simulink model "receiver_overall_v3"  (Simulink 7.5)
settings: Solver=FixedStepDiscrete  SolverMode=SingleTasking  StartTime=0.0  StopTime=(length(simin.signals.values)-1)/Fs  FixedStep=1  RelTol=1e-3
undefined symbols (not defined in the file): Fs
libraries: xbsIndex_r4 x939, symbols x8, dspsigops x2
(part 5 of 9)

== system receiver_overall_v3/Receiver/FM demod/AGC/CORDIC DIVIDER/Iterative Divider/CORDIC PE7 ==
  note: X = x - y if y < 0, otherwise
      |    = x + y
      | Y = y + x if y < 0, otherwise
      |    = y - x
      | Z = z - atan(1/2^i) if y < 0, otherwise
      |    = z + atan(1/2^i)
  x : Inport  OutDataType=sfix(16)  OutScaling=2^0
  y : Inport  Port=2  OutDataType=sfix(16)  OutScaling=2^0
  z : Inport  Port=3  OutDataType=sfix(16)  OutScaling=2^0
  AddSub1 : xbsIndex_r4/AddSub  mode=Addition or Subtraction  use_carryin=off  use_carryout=off  en=off  latency=pipeline  precision=User Defined  arith_type="Signed  (2's comp)"  n_bits=pe_nbits  bin_pt=pe_binpt  quantization=Truncate  overflow=Wrap  dbl_ovrd=off  use_behavioral_HDL=on  hw_selection=Fabric  pipelined=off  use_rpm=off  block_type=addsub
      settings: xl_area=[8 16 0 16 0 0 0]  block_version=VER_STRING_GOES_HERE
  AddSub2 : xbsIndex_r4/AddSub  mode=Addition or Subtraction  use_carryin=off  use_carryout=off  en=off  latency=pipeline  precision=User Defined  arith_type="Signed  (2's comp)"  n_bits=stages+2  bin_pt=stages  quantization=Truncate  overflow=Wrap  dbl_ovrd=off  use_behavioral_HDL=on  hw_selection=Fabric  pipelined=off  use_rpm=off  block_type=addsub
      settings: xl_area=[8 16 0 16 0 0 0]  block_version=VER_STRING_GOES_HERE
  Constant : xbsIndex_r4/Constant  arith_type=Signed (2's comp)  const=2^-ii  n_bits=stages+2  bin_pt=stages  explicit_period=off  period=1  equ=P=C  opselect=C  inp2=PCIN>>17  opr=+  inp1=P  carry=CIN  dbl_ovrd=off  block_type=constant
      settings: block_version=VER_STRING_GOES_HERE
  Inverter : xbsIndex_r4/Inverter  en=off  latency=0  dbl_ovrd=off  block_type=inv
      settings: xl_area=[1 0 0 1 0 0 0]  block_version=VER_STRING_GOES_HERE
  Register : xbsIndex_r4/Register  init=0  rst=off  en=off  dbl_ovrd=off  block_type=register
      settings: xl_area=[8 16 0 0 0 0 0]  block_version=VER_STRING_GOES_HERE
  Shift : xbsIndex_r4/Shift  shift_dir=Right  shift_bits=ii  en=off  latency=0  precision=User Defined  arith_type="Signed  (2's comp)"  n_bits=pe_nbits  bin_pt=pe_binpt  quantization=Truncate  overflow=Wrap  dbl_ovrd=off  block_type=shift
      settings: xl_area=[0 0 0 0 0 0 0]  block_version=VER_STRING_GOES_HERE
  Slice : xbsIndex_r4/Slice  nbits=1  boolean_output=on  mode=Upper Bit Location + Width  bit1=0  base1=MSB of Input  bit0=0  base0=LSB of Input  dbl_ovrd=off  block_type=slice
      settings: infoedit="Extracts a given range of bits from each input sample and presents it at the output.  The output type is ordinarily unsigned with binary point at zero, but can be Boolean when the slice is one bit wide.<P><P>Hardware notes: In hardware this block costs nothing."  block_version=VER_STRING_GOES_HERE
  X : Outport  OutDataType=sfix(16)  OutScaling=2^0
  Y : Outport  Port=2  OutDataType=sfix(16)  OutScaling=2^0
  Z : Outport  Port=3  OutDataType=sfix(16)  OutScaling=2^0
  wires:
  Register/1 -> X/1
  x/1 -> Register/1, Shift/1
  y/1 -> AddSub1/1, Slice/1
  z/1 -> AddSub2/1
  AddSub1/1 -> Y/1
  AddSub2/1 -> Z/1
  Constant/1 -> AddSub2/2
  Inverter/1 -> AddSub1/3
  Shift/1 -> AddSub1/2
  Slice/1 -> AddSub2/3, Inverter/1

== system receiver_overall_v3/Receiver/FM demod/AGC/CORDIC DIVIDER/Iterative Divider/CORDIC PE8 ==
  note: X = x - y if y < 0, otherwise
      |    = x + y
      | Y = y + x if y < 0, otherwise
      |    = y - x
      | Z = z - atan(1/2^i) if y < 0, otherwise
      |    = z + atan(1/2^i)
  x : Inport  OutDataType=sfix(16)  OutScaling=2^0
  y : Inport  Port=2  OutDataType=sfix(16)  OutScaling=2^0
  z : Inport  Port=3  OutDataType=sfix(16)  OutScaling=2^0
  AddSub1 : xbsIndex_r4/AddSub  mode=Addition or Subtraction  use_carryin=off  use_carryout=off  en=off  latency=pipeline  precision=User Defined  arith_type="Signed  (2's comp)"  n_bits=pe_nbits  bin_pt=pe_binpt  quantization=Truncate  overflow=Wrap  dbl_ovrd=off  use_behavioral_HDL=on  hw_selection=Fabric  pipelined=off  use_rpm=off  block_type=addsub
      settings: xl_area=[8 16 0 16 0 0 0]  block_version=VER_STRING_GOES_HERE
  AddSub2 : xbsIndex_r4/AddSub  mode=Addition or Subtraction  use_carryin=off  use_carryout=off  en=off  latency=pipeline  precision=User Defined  arith_type="Signed  (2's comp)"  n_bits=stages+2  bin_pt=stages  quantization=Truncate  overflow=Wrap  dbl_ovrd=off  use_behavioral_HDL=on  hw_selection=Fabric  pipelined=off  use_rpm=off  block_type=addsub
      settings: xl_area=[8 16 0 16 0 0 0]  block_version=VER_STRING_GOES_HERE
  Constant : xbsIndex_r4/Constant  arith_type=Signed (2's comp)  const=2^-ii  n_bits=stages+2  bin_pt=stages  explicit_period=off  period=1  equ=P=C  opselect=C  inp2=PCIN>>17  opr=+  inp1=P  carry=CIN  dbl_ovrd=off  block_type=constant
      settings: block_version=VER_STRING_GOES_HERE
  Inverter : xbsIndex_r4/Inverter  en=off  latency=0  dbl_ovrd=off  block_type=inv
      settings: xl_area=[1 0 0 1 0 0 0]  block_version=VER_STRING_GOES_HERE
  Register : xbsIndex_r4/Register  init=0  rst=off  en=off  dbl_ovrd=off  block_type=register
      settings: xl_area=[8 16 0 0 0 0 0]  block_version=VER_STRING_GOES_HERE
  Shift : xbsIndex_r4/Shift  shift_dir=Right  shift_bits=ii  en=off  latency=0  precision=User Defined  arith_type="Signed  (2's comp)"  n_bits=pe_nbits  bin_pt=pe_binpt  quantization=Truncate  overflow=Wrap  dbl_ovrd=off  block_type=shift
      settings: xl_area=[0 0 0 0 0 0 0]  block_version=VER_STRING_GOES_HERE
  Slice : xbsIndex_r4/Slice  nbits=1  boolean_output=on  mode=Upper Bit Location + Width  bit1=0  base1=MSB of Input  bit0=0  base0=LSB of Input  dbl_ovrd=off  block_type=slice
      settings: infoedit="Extracts a given range of bits from each input sample and presents it at the output.  The output type is ordinarily unsigned with binary point at zero, but can be Boolean when the slice is one bit wide.<P><P>Hardware notes: In hardware this block costs nothing."  block_version=VER_STRING_GOES_HERE
  X : Outport  OutDataType=sfix(16)  OutScaling=2^0
  Y : Outport  Port=2  OutDataType=sfix(16)  OutScaling=2^0
  Z : Outport  Port=3  OutDataType=sfix(16)  OutScaling=2^0
  wires:
  Register/1 -> X/1
  x/1 -> Register/1, Shift/1
  y/1 -> AddSub1/1, Slice/1
  z/1 -> AddSub2/1
  AddSub1/1 -> Y/1
  AddSub2/1 -> Z/1
  Constant/1 -> AddSub2/2
  Inverter/1 -> AddSub1/3
  Shift/1 -> AddSub1/2
  Slice/1 -> AddSub2/3, Inverter/1

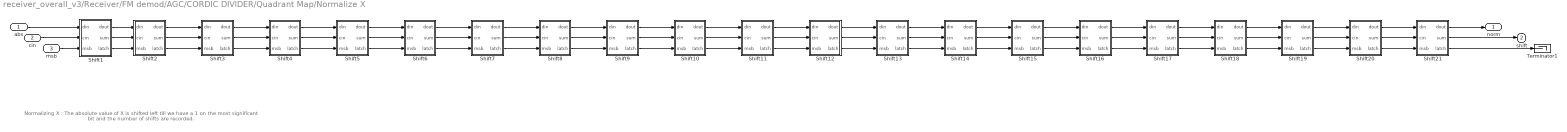
== system receiver_overall_v3/Receiver/FM demod/AGC/CORDIC DIVIDER/Quadrant Map/Normalize X ==
  note: Normalizing X : The absolute value of X is shifted left till we have a 1
      | on the most significant bit and the number of shifts are recorded.
  abs : Inport  OutDataType=sfix(16)  OutScaling=2^0
  cin : Inport  Port=2  OutDataType=sfix(16)  OutScaling=2^0
  msb : Inport  Port=3  OutDataType=sfix(16)  OutScaling=2^0
  Shift1 : Subsystem  mask(Normalize Shift Stage){num_bits=num_bits, bin_point=bin_point}
      mask prompts: num_bits "Number of Bits"; bin_point "Binary Point Position"
      mask init:
      | [bg,fg] = xlcmap('XBlock',0);
      | iPos = get_param(gcb,'Position');
      | iWidth=iPos(3)-iPos(1); iHeight=iPos(4)-iPos(2);
      | iCx=iWidth/2;
      | iCy=iHeight/2;
      | [logoX, logoY] = xlogo(iPos);
      mask Display:
      | patch([0 iWidth iWidth 0],[0 0 iHeight iHeight] , bg);
      | patch(logoX,logoY , fg);
      | port_label('input',1,'din');
      | port_label('input',2,'cin');
      | port_label('input',3,'msb');
      | port_label('output',1,'dout');
      | port_label('output',2,'sum');
      | port_label('output',3,'latch');
      | plot([0 0 iWidth iWidth 0], [0 iHeight iHeight 0 0]);
  Shift10 : Subsystem  mask(Normalize Shift Stage){num_bits=num_bits, bin_point=bin_point}
      mask prompts: num_bits "Number of Bits"; bin_point "Binary Point Position"
      mask init:
      | [bg,fg] = xlcmap('XBlock',0);
      | iPos = get_param(gcb,'Position');
      | iWidth=iPos(3)-iPos(1); iHeight=iPos(4)-iPos(2);
      | iCx=iWidth/2;
      | iCy=iHeight/2;
      | [logoX, logoY] = xlogo(iPos);
      mask Display:
      | patch([0 iWidth iWidth 0],[0 0 iHeight iHeight] , bg);
      | patch(logoX,logoY , fg);
      | port_label('input',1,'din');
      | port_label('input',2,'cin');
      | port_label('input',3,'msb');
      | port_label('output',1,'dout');
      | port_label('output',2,'sum');
      | port_label('output',3,'latch');
      | plot([0 0 iWidth iWidth 0], [0 iHeight iHeight 0 0]);
  Shift11 : Subsystem  mask(Normalize Shift Stage){num_bits=num_bits, bin_point=bin_point}
      mask prompts: num_bits "Number of Bits"; bin_point "Binary Point Position"
      mask init:
      | [bg,fg] = xlcmap('XBlock',0);
      | iPos = get_param(gcb,'Position');
      | iWidth=iPos(3)-iPos(1); iHeight=iPos(4)-iPos(2);
      | iCx=iWidth/2;
      | iCy=iHeight/2;
      | [logoX, logoY] = xlogo(iPos);
      mask Display:
      | patch([0 iWidth iWidth 0],[0 0 iHeight iHeight] , bg);
      | patch(logoX,logoY , fg);
      | port_label('input',1,'din');
      | port_label('input',2,'cin');
      | port_label('input',3,'msb');
      | port_label('output',1,'dout');
      | port_label('output',2,'sum');
      | port_label('output',3,'latch');
      | plot([0 0 iWidth iWidth 0], [0 iHeight iHeight 0 0]);
  Shift12 : Subsystem  mask(Normalize Shift Stage){num_bits=num_bits, bin_point=bin_point}
      mask prompts: num_bits "Number of Bits"; bin_point "Binary Point Position"
      mask init:
      | [bg,fg] = xlcmap('XBlock',0);
      | iPos = get_param(gcb,'Position');
      | iWidth=iPos(3)-iPos(1); iHeight=iPos(4)-iPos(2);
      | iCx=iWidth/2;
      | iCy=iHeight/2;
      | [logoX, logoY] = xlogo(iPos);
      mask Display:
      | patch([0 iWidth iWidth 0],[0 0 iHeight iHeight] , bg);
      | patch(logoX,logoY , fg);
      | port_label('input',1,'din');
      | port_label('input',2,'cin');
      | port_label('input',3,'msb');
      | port_label('output',1,'dout');
      | port_label('output',2,'sum');
      | port_label('output',3,'latch');
      | plot([0 0 iWidth iWidth 0], [0 iHeight iHeight 0 0]);
  Shift13 : Subsystem  mask(Normalize Shift Stage){num_bits=num_bits, bin_point=bin_point}
      mask prompts: num_bits "Number of Bits"; bin_point "Binary Point Position"
      mask init:
      | [bg,fg] = xlcmap('XBlock',0);
      | iPos = get_param(gcb,'Position');
      | iWidth=iPos(3)-iPos(1); iHeight=iPos(4)-iPos(2);
      | iCx=iWidth/2;
      | iCy=iHeight/2;
      | [logoX, logoY] = xlogo(iPos);
      mask Display:
      | patch([0 iWidth iWidth 0],[0 0 iHeight iHeight] , bg);
      | patch(logoX,logoY , fg);
      | port_label('input',1,'din');
      | port_label('input',2,'cin');
      | port_label('input',3,'msb');
      | port_label('output',1,'dout');
      | port_label('output',2,'sum');
      | port_label('output',3,'latch');
      | plot([0 0 iWidth iWidth 0], [0 iHeight iHeight 0 0]);
  Shift14 : Subsystem  mask(Normalize Shift Stage){num_bits=num_bits, bin_point=bin_point}
      mask prompts: num_bits "Number of Bits"; bin_point "Binary Point Position"
      mask init:
      | [bg,fg] = xlcmap('XBlock',0);
      | iPos = get_param(gcb,'Position');
      | iWidth=iPos(3)-iPos(1); iHeight=iPos(4)-iPos(2);
      | iCx=iWidth/2;
      | iCy=iHeight/2;
      | [logoX, logoY] = xlogo(iPos);
      mask Display:
      | patch([0 iWidth iWidth 0],[0 0 iHeight iHeight] , bg);
      | patch(logoX,logoY , fg);
      | port_label('input',1,'din');
      | port_label('input',2,'cin');
      | port_label('input',3,'msb');
      | port_label('output',1,'dout');
      | port_label('output',2,'sum');
      | port_label('output',3,'latch');
      | plot([0 0 iWidth iWidth 0], [0 iHeight iHeight 0 0]);
  Shift15 : Subsystem  mask(Normalize Shift Stage){num_bits=num_bits, bin_point=bin_point}
      mask prompts: num_bits "Number of Bits"; bin_point "Binary Point Position"
      mask init:
      | [bg,fg] = xlcmap('XBlock',0);
      | iPos = get_param(gcb,'Position');
      | iWidth=iPos(3)-iPos(1); iHeight=iPos(4)-iPos(2);
      | iCx=iWidth/2;
      | iCy=iHeight/2;
      | [logoX, logoY] = xlogo(iPos);
      mask Display:
      | patch([0 iWidth iWidth 0],[0 0 iHeight iHeight] , bg);
      | patch(logoX,logoY , fg);
      | port_label('input',1,'din');
      | port_label('input',2,'cin');
      | port_label('input',3,'msb');
      | port_label('output',1,'dout');
      | port_label('output',2,'sum');
      | port_label('output',3,'latch');
      | plot([0 0 iWidth iWidth 0], [0 iHeight iHeight 0 0]);
  Shift16 : Subsystem  mask(Normalize Shift Stage){num_bits=num_bits, bin_point=bin_point}
      mask prompts: num_bits "Number of Bits"; bin_point "Binary Point Position"
      mask init:
      | [bg,fg] = xlcmap('XBlock',0);
      | iPos = get_param(gcb,'Position');
      | iWidth=iPos(3)-iPos(1); iHeight=iPos(4)-iPos(2);
      | iCx=iWidth/2;
      | iCy=iHeight/2;
      | [logoX, logoY] = xlogo(iPos);
      mask Display:
      | patch([0 iWidth iWidth 0],[0 0 iHeight iHeight] , bg);
      | patch(logoX,logoY , fg);
      | port_label('input',1,'din');
      | port_label('input',2,'cin');
      | port_label('input',3,'msb');
      | port_label('output',1,'dout');
      | port_label('output',2,'sum');
      | port_label('output',3,'latch');
      | plot([0 0 iWidth iWidth 0], [0 iHeight iHeight 0 0]);
  Shift17 : Subsystem  mask(Normalize Shift Stage){num_bits=num_bits, bin_point=bin_point}
      mask prompts: num_bits "Number of Bits"; bin_point "Binary Point Position"
      mask init:
      | [bg,fg] = xlcmap('XBlock',0);
      | iPos = get_param(gcb,'Position');
      | iWidth=iPos(3)-iPos(1); iHeight=iPos(4)-iPos(2);
      | iCx=iWidth/2;
      | iCy=iHeight/2;
      | [logoX, logoY] = xlogo(iPos);
      mask Display:
      | patch([0 iWidth iWidth 0],[0 0 iHeight iHeight] , bg);
      | patch(logoX,logoY , fg);
      | port_label('input',1,'din');
      | port_label('input',2,'cin');
      | port_label('input',3,'msb');
      | port_label('output',1,'dout');
      | port_label('output',2,'sum');
      | port_label('output',3,'latch');
      | plot([0 0 iWidth iWidth 0], [0 iHeight iHeight 0 0]);
  Shift18 : Subsystem  mask(Normalize Shift Stage){num_bits=num_bits, bin_point=bin_point}
      mask prompts: num_bits "Number of Bits"; bin_point "Binary Point Position"
      mask init:
      | [bg,fg] = xlcmap('XBlock',0);
      | iPos = get_param(gcb,'Position');
      | iWidth=iPos(3)-iPos(1); iHeight=iPos(4)-iPos(2);
      | iCx=iWidth/2;
      | iCy=iHeight/2;
      | [logoX, logoY] = xlogo(iPos);
      mask Display:
      | patch([0 iWidth iWidth 0],[0 0 iHeight iHeight] , bg);
      | patch(logoX,logoY , fg);
      | port_label('input',1,'din');
      | port_label('input',2,'cin');
      | port_label('input',3,'msb');
      | port_label('output',1,'dout');
      | port_label('output',2,'sum');
      | port_label('output',3,'latch');
      | plot([0 0 iWidth iWidth 0], [0 iHeight iHeight 0 0]);
  Shift19 : Subsystem  mask(Normalize Shift Stage){num_bits=num_bits, bin_point=bin_point}
      mask prompts: num_bits "Number of Bits"; bin_point "Binary Point Position"
      mask init:
      | [bg,fg] = xlcmap('XBlock',0);
      | iPos = get_param(gcb,'Position');
      | iWidth=iPos(3)-iPos(1); iHeight=iPos(4)-iPos(2);
      | iCx=iWidth/2;
      | iCy=iHeight/2;
      | [logoX, logoY] = xlogo(iPos);
      mask Display:
      | patch([0 iWidth iWidth 0],[0 0 iHeight iHeight] , bg);
      | patch(logoX,logoY , fg);
      | port_label('input',1,'din');
      | port_label('input',2,'cin');
      | port_label('input',3,'msb');
      | port_label('output',1,'dout');
      | port_label('output',2,'sum');
      | port_label('output',3,'latch');
      | plot([0 0 iWidth iWidth 0], [0 iHeight iHeight 0 0]);
  Shift2 : Subsystem  mask(Normalize Shift Stage){num_bits=num_bits, bin_point=bin_point}
      mask prompts: num_bits "Number of Bits"; bin_point "Binary Point Position"
      mask init:
      | [bg,fg] = xlcmap('XBlock',0);
      | iPos = get_param(gcb,'Position');
      | iWidth=iPos(3)-iPos(1); iHeight=iPos(4)-iPos(2);
      | iCx=iWidth/2;
      | iCy=iHeight/2;
      | [logoX, logoY] = xlogo(iPos);
      mask Display:
      | patch([0 iWidth iWidth 0],[0 0 iHeight iHeight] , bg);
      | patch(logoX,logoY , fg);
      | port_label('input',1,'din');
      | port_label('input',2,'cin');
      | port_label('input',3,'msb');
      | port_label('output',1,'dout');
      | port_label('output',2,'sum');
      | port_label('output',3,'latch');
      | plot([0 0 iWidth iWidth 0], [0 iHeight iHeight 0 0]);
  Shift20 : Subsystem  mask(Normalize Shift Stage){num_bits=num_bits, bin_point=bin_point}
      mask prompts: num_bits "Number of Bits"; bin_point "Binary Point Position"
      mask init:
      | [bg,fg] = xlcmap('XBlock',0);
      | iPos = get_param(gcb,'Position');
      | iWidth=iPos(3)-iPos(1); iHeight=iPos(4)-iPos(2);
      | iCx=iWidth/2;
      | iCy=iHeight/2;
      | [logoX, logoY] = xlogo(iPos);
      mask Display:
      | patch([0 iWidth iWidth 0],[0 0 iHeight iHeight] , bg);
      | patch(logoX,logoY , fg);
      | port_label('input',1,'din');
      | port_label('input',2,'cin');
      | port_label('input',3,'msb');
      | port_label('output',1,'dout');
      | port_label('output',2,'sum');
      | port_label('output',3,'latch');
      | plot([0 0 iWidth iWidth 0], [0 iHeight iHeight 0 0]);
  Shift21 : Subsystem  mask(Normalize Shift Stage){num_bits=num_bits, bin_point=bin_point}
      mask prompts: num_bits "Number of Bits"; bin_point "Binary Point Position"
      mask init:
      | [bg,fg] = xlcmap('XBlock',0);
      | iPos = get_param(gcb,'Position');
      | iWidth=iPos(3)-iPos(1); iHeight=iPos(4)-iPos(2);
      | iCx=iWidth/2;
      | iCy=iHeight/2;
      | [logoX, logoY] = xlogo(iPos);
      mask Display:
      | patch([0 iWidth iWidth 0],[0 0 iHeight iHeight] , bg);
      | patch(logoX,logoY , fg);
      | port_label('input',1,'din');
      | port_label('input',2,'cin');
      | port_label('input',3,'msb');
      | port_label('output',1,'dout');
      | port_label('output',2,'sum');
      | port_label('output',3,'latch');
      | plot([0 0 iWidth iWidth 0], [0 iHeight iHeight 0 0]);
  Shift3 : Subsystem  mask(Normalize Shift Stage){num_bits=num_bits, bin_point=bin_point}
      mask prompts: num_bits "Number of Bits"; bin_point "Binary Point Position"
      mask init:
      | [bg,fg] = xlcmap('XBlock',0);
      | iPos = get_param(gcb,'Position');
      | iWidth=iPos(3)-iPos(1); iHeight=iPos(4)-iPos(2);
      | iCx=iWidth/2;
      | iCy=iHeight/2;
      | [logoX, logoY] = xlogo(iPos);
      mask Display:
      | patch([0 iWidth iWidth 0],[0 0 iHeight iHeight] , bg);
      | patch(logoX,logoY , fg);
      | port_label('input',1,'din');
      | port_label('input',2,'cin');
      | port_label('input',3,'msb');
      | port_label('output',1,'dout');
      | port_label('output',2,'sum');
      | port_label('output',3,'latch');
      | plot([0 0 iWidth iWidth 0], [0 iHeight iHeight 0 0]);
  Shift4 : Subsystem  mask(Normalize Shift Stage){num_bits=num_bits, bin_point=bin_point}
      mask prompts: num_bits "Number of Bits"; bin_point "Binary Point Position"
      mask init:
      | [bg,fg] = xlcmap('XBlock',0);
      | iPos = get_param(gcb,'Position');
      | iWidth=iPos(3)-iPos(1); iHeight=iPos(4)-iPos(2);
      | iCx=iWidth/2;
      | iCy=iHeight/2;
      | [logoX, logoY] = xlogo(iPos);
      mask Display:
      | patch([0 iWidth iWidth 0],[0 0 iHeight iHeight] , bg);
      | patch(logoX,logoY , fg);
      | port_label('input',1,'din');
      | port_label('input',2,'cin');
      | port_label('input',3,'msb');
      | port_label('output',1,'dout');
      | port_label('output',2,'sum');
      | port_label('output',3,'latch');
      | plot([0 0 iWidth iWidth 0], [0 iHeight iHeight 0 0]);
  Shift5 : Subsystem  mask(Normalize Shift Stage){num_bits=num_bits, bin_point=bin_point}
      mask prompts: num_bits "Number of Bits"; bin_point "Binary Point Position"
      mask init:
      | [bg,fg] = xlcmap('XBlock',0);
      | iPos = get_param(gcb,'Position');
      | iWidth=iPos(3)-iPos(1); iHeight=iPos(4)-iPos(2);
      | iCx=iWidth/2;
      | iCy=iHeight/2;
      | [logoX, logoY] = xlogo(iPos);
      mask Display:
      | patch([0 iWidth iWidth 0],[0 0 iHeight iHeight] , bg);
      | patch(logoX,logoY , fg);
      | port_label('input',1,'din');
      | port_label('input',2,'cin');
      | port_label('input',3,'msb');
      | port_label('output',1,'dout');
      | port_label('output',2,'sum');
      | port_label('output',3,'latch');
      | plot([0 0 iWidth iWidth 0], [0 iHeight iHeight 0 0]);
  Shift6 : Subsystem  mask(Normalize Shift Stage){num_bits=num_bits, bin_point=bin_point}
      mask prompts: num_bits "Number of Bits"; bin_point "Binary Point Position"
      mask init:
      | [bg,fg] = xlcmap('XBlock',0);
      | iPos = get_param(gcb,'Position');
      | iWidth=iPos(3)-iPos(1); iHeight=iPos(4)-iPos(2);
      | iCx=iWidth/2;
      | iCy=iHeight/2;
      | [logoX, logoY] = xlogo(iPos);
      mask Display:
      | patch([0 iWidth iWidth 0],[0 0 iHeight iHeight] , bg);
      | patch(logoX,logoY , fg);
      | port_label('input',1,'din');
      | port_label('input',2,'cin');
      | port_label('input',3,'msb');
      | port_label('output',1,'dout');
      | port_label('output',2,'sum');
      | port_label('output',3,'latch');
      | plot([0 0 iWidth iWidth 0], [0 iHeight iHeight 0 0]);
  Shift7 : Subsystem  mask(Normalize Shift Stage){num_bits=num_bits, bin_point=bin_point}
      mask prompts: num_bits "Number of Bits"; bin_point "Binary Point Position"
      mask init:
      | [bg,fg] = xlcmap('XBlock',0);
      | iPos = get_param(gcb,'Position');
      | iWidth=iPos(3)-iPos(1); iHeight=iPos(4)-iPos(2);
      | iCx=iWidth/2;
      | iCy=iHeight/2;
      | [logoX, logoY] = xlogo(iPos);
      mask Display:
      | patch([0 iWidth iWidth 0],[0 0 iHeight iHeight] , bg);
      | patch(logoX,logoY , fg);
      | port_label('input',1,'din');
      | port_label('input',2,'cin');
      | port_label('input',3,'msb');
      | port_label('output',1,'dout');
      | port_label('output',2,'sum');
      | port_label('output',3,'latch');
      | plot([0 0 iWidth iWidth 0], [0 iHeight iHeight 0 0]);
  Shift8 : Subsystem  mask(Normalize Shift Stage){num_bits=num_bits, bin_point=bin_point}
      mask prompts: num_bits "Number of Bits"; bin_point "Binary Point Position"
      mask init:
      | [bg,fg] = xlcmap('XBlock',0);
      | iPos = get_param(gcb,'Position');
      | iWidth=iPos(3)-iPos(1); iHeight=iPos(4)-iPos(2);
      | iCx=iWidth/2;
      | iCy=iHeight/2;
      | [logoX, logoY] = xlogo(iPos);
      mask Display:
      | patch([0 iWidth iWidth 0],[0 0 iHeight iHeight] , bg);
      | patch(logoX,logoY , fg);
      | port_label('input',1,'din');
      | port_label('input',2,'cin');
      | port_label('input',3,'msb');
      | port_label('output',1,'dout');
      | port_label('output',2,'sum');
      | port_label('output',3,'latch');
      | plot([0 0 iWidth iWidth 0], [0 iHeight iHeight 0 0]);
  Shift9 : Subsystem  mask(Normalize Shift Stage){num_bits=num_bits, bin_point=bin_point}
      mask prompts: num_bits "Number of Bits"; bin_point "Binary Point Position"
      mask init:
      | [bg,fg] = xlcmap('XBlock',0);
      | iPos = get_param(gcb,'Position');
      | iWidth=iPos(3)-iPos(1); iHeight=iPos(4)-iPos(2);
      | iCx=iWidth/2;
      | iCy=iHeight/2;
      | [logoX, logoY] = xlogo(iPos);
      mask Display:
      | patch([0 iWidth iWidth 0],[0 0 iHeight iHeight] , bg);
      | patch(logoX,logoY , fg);
      | port_label('input',1,'din');
      | port_label('input',2,'cin');
      | port_label('input',3,'msb');
      | port_label('output',1,'dout');
      | port_label('output',2,'sum');
      | port_label('output',3,'latch');
      | plot([0 0 iWidth iWidth 0], [0 iHeight iHeight 0 0]);
  Terminator1 : Terminator
  norm : Outport  OutDataType=sfix(16)  OutScaling=2^0
  shift : Outport  Port=2  OutDataType=sfix(16)  OutScaling=2^0
  wires:
  abs/1 -> Shift1/1(din)
  cin/1 -> Shift1/2(cin)
  msb/1 -> Shift1/3(msb)
  Shift1/1(dout) -> Shift2/1(din)
  Shift1/2(sum) -> Shift2/2(cin)
  Shift1/3(latch) -> Shift2/3(msb)
  Shift2/1(dout) -> Shift3/1(din)
  Shift2/2(sum) -> Shift3/2(cin)
  Shift2/3(latch) -> Shift3/3(msb)
  Shift3/1(dout) -> Shift4/1(din)
  Shift3/2(sum) -> Shift4/2(cin)
  Shift3/3(latch) -> Shift4/3(msb)
  Shift4/1(dout) -> Shift5/1(din)
  Shift4/2(sum) -> Shift5/2(cin)
  Shift4/3(latch) -> Shift5/3(msb)
  Shift5/1(dout) -> Shift6/1(din)
  Shift5/2(sum) -> Shift6/2(cin)
  Shift5/3(latch) -> Shift6/3(msb)
  Shift6/1(dout) -> Shift7/1(din)
  Shift6/2(sum) -> Shift7/2(cin)
  Shift6/3(latch) -> Shift7/3(msb)
  Shift7/1(dout) -> Shift8/1(din)
  Shift7/2(sum) -> Shift8/2(cin)
  Shift7/3(latch) -> Shift8/3(msb)
  Shift8/1(dout) -> Shift9/1(din)
  Shift8/2(sum) -> Shift9/2(cin)
  Shift8/3(latch) -> Shift9/3(msb)
  Shift9/1(dout) -> Shift10/1(din)
  Shift9/2(sum) -> Shift10/2(cin)
  Shift9/3(latch) -> Shift10/3(msb)
  Shift10/1(dout) -> Shift11/1(din)
  Shift10/2(sum) -> Shift11/2(cin)
  Shift10/3(latch) -> Shift11/3(msb)
  Shift11/1(dout) -> Shift12/1(din)
  Shift11/2(sum) -> Shift12/2(cin)
  Shift11/3(latch) -> Shift12/3(msb)
  Shift12/1(dout) -> Shift13/1(din)
  Shift12/2(sum) -> Shift13/2(cin)
  Shift12/3(latch) -> Shift13/3(msb)
  Shift13/1(dout) -> Shift14/1(din)
  Shift13/2(sum) -> Shift14/2(cin)
  Shift13/3(latch) -> Shift14/3(msb)
  Shift14/1(dout) -> Shift15/1(din)
  Shift14/2(sum) -> Shift15/2(cin)
  Shift14/3(latch) -> Shift15/3(msb)
  Shift15/1(dout) -> Shift16/1(din)
  Shift15/2(sum) -> Shift16/2(cin)
  Shift15/3(latch) -> Shift16/3(msb)
  Shift16/1(dout) -> Shift17/1(din)
  Shift16/2(sum) -> Shift17/2(cin)
  Shift16/3(latch) -> Shift17/3(msb)
  Shift17/1(dout) -> Shift18/1(din)
  Shift17/2(sum) -> Shift18/2(cin)
  Shift17/3(latch) -> Shift18/3(msb)
  Shift18/1(dout) -> Shift19/1(din)
  Shift18/2(sum) -> Shift19/2(cin)
  Shift18/3(latch) -> Shift19/3(msb)
  Shift19/1(dout) -> Shift20/1(din)
  Shift19/2(sum) -> Shift20/2(cin)
  Shift19/3(latch) -> Shift20/3(msb)
  Shift20/1(dout) -> Shift21/1(din)
  Shift20/2(sum) -> Shift21/2(cin)
  Shift20/3(latch) -> Shift21/3(msb)
  Shift21/1(dout) -> norm/1
  Shift21/2(sum) -> shift/1
  Shift21/3(latch) -> Terminator1/1

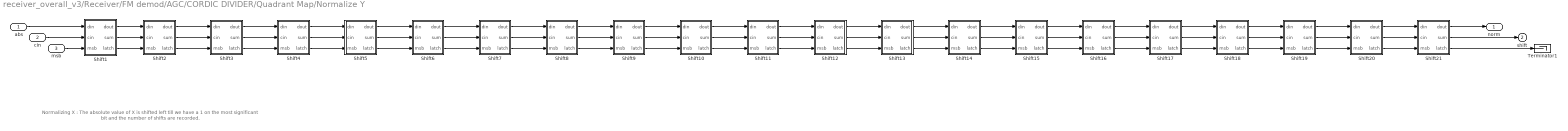
== system receiver_overall_v3/Receiver/FM demod/AGC/CORDIC DIVIDER/Quadrant Map/Normalize Y ==
  note: Normalizing X : The absolute value of X is shifted left till we have a 1
      | on the most significant bit and the number of shifts are recorded.
  abs : Inport  OutDataType=sfix(16)  OutScaling=2^0
  cin : Inport  Port=2  OutDataType=sfix(16)  OutScaling=2^0
  msb : Inport  Port=3  OutDataType=sfix(16)  OutScaling=2^0
  Shift1 : Subsystem  mask(Normalize Shift Stage){num_bits=num_bits, bin_point=bin_point}
      mask prompts: num_bits "Number of Bits"; bin_point "Binary Point Position"
      mask init:
      | [bg,fg] = xlcmap('XBlock',0);
      | iPos = get_param(gcb,'Position');
      | iWidth=iPos(3)-iPos(1); iHeight=iPos(4)-iPos(2);
      | iCx=iWidth/2;
      | iCy=iHeight/2;
      | [logoX, logoY] = xlogo(iPos);
      mask Display:
      | patch([0 iWidth iWidth 0],[0 0 iHeight iHeight] , bg);
      | patch(logoX,logoY , fg);
      | port_label('input',1,'din');
      | port_label('input',2,'cin');
      | port_label('input',3,'msb');
      | port_label('output',1,'dout');
      | port_label('output',2,'sum');
      | port_label('output',3,'latch');
      | plot([0 0 iWidth iWidth 0], [0 iHeight iHeight 0 0]);
  Shift10 : Subsystem  mask(Normalize Shift Stage){num_bits=num_bits, bin_point=bin_point}
      mask prompts: num_bits "Number of Bits"; bin_point "Binary Point Position"
      mask init:
      | [bg,fg] = xlcmap('XBlock',0);
      | iPos = get_param(gcb,'Position');
      | iWidth=iPos(3)-iPos(1); iHeight=iPos(4)-iPos(2);
      | iCx=iWidth/2;
      | iCy=iHeight/2;
      | [logoX, logoY] = xlogo(iPos);
      mask Display:
      | patch([0 iWidth iWidth 0],[0 0 iHeight iHeight] , bg);
      | patch(logoX,logoY , fg);
      | port_label('input',1,'din');
      | port_label('input',2,'cin');
      | port_label('input',3,'msb');
      | port_label('output',1,'dout');
      | port_label('output',2,'sum');
      | port_label('output',3,'latch');
      | plot([0 0 iWidth iWidth 0], [0 iHeight iHeight 0 0]);
  Shift11 : Subsystem  mask(Normalize Shift Stage){num_bits=num_bits, bin_point=bin_point}
      mask prompts: num_bits "Number of Bits"; bin_point "Binary Point Position"
      mask init:
      | [bg,fg] = xlcmap('XBlock',0);
      | iPos = get_param(gcb,'Position');
      | iWidth=iPos(3)-iPos(1); iHeight=iPos(4)-iPos(2);
      | iCx=iWidth/2;
      | iCy=iHeight/2;
      | [logoX, logoY] = xlogo(iPos);
      mask Display:
      | patch([0 iWidth iWidth 0],[0 0 iHeight iHeight] , bg);
      | patch(logoX,logoY , fg);
      | port_label('input',1,'din');
      | port_label('input',2,'cin');
      | port_label('input',3,'msb');
      | port_label('output',1,'dout');
      | port_label('output',2,'sum');
      | port_label('output',3,'latch');
      | plot([0 0 iWidth iWidth 0], [0 iHeight iHeight 0 0]);
  Shift12 : Subsystem  mask(Normalize Shift Stage){num_bits=num_bits, bin_point=bin_point}
      mask prompts: num_bits "Number of Bits"; bin_point "Binary Point Position"
      mask init:
      | [bg,fg] = xlcmap('XBlock',0);
      | iPos = get_param(gcb,'Position');
      | iWidth=iPos(3)-iPos(1); iHeight=iPos(4)-iPos(2);
      | iCx=iWidth/2;
      | iCy=iHeight/2;
      | [logoX, logoY] = xlogo(iPos);
      mask Display:
      | patch([0 iWidth iWidth 0],[0 0 iHeight iHeight] , bg);
      | patch(logoX,logoY , fg);
      | port_label('input',1,'din');
      | port_label('input',2,'cin');
      | port_label('input',3,'msb');
      | port_label('output',1,'dout');
      | port_label('output',2,'sum');
      | port_label('output',3,'latch');
      | plot([0 0 iWidth iWidth 0], [0 iHeight iHeight 0 0]);
  Shift13 : Subsystem  mask(Normalize Shift Stage){num_bits=num_bits, bin_point=bin_point}
      mask prompts: num_bits "Number of Bits"; bin_point "Binary Point Position"
      mask init:
      | [bg,fg] = xlcmap('XBlock',0);
      | iPos = get_param(gcb,'Position');
      | iWidth=iPos(3)-iPos(1); iHeight=iPos(4)-iPos(2);
      | iCx=iWidth/2;
      | iCy=iHeight/2;
      | [logoX, logoY] = xlogo(iPos);
      mask Display:
      | patch([0 iWidth iWidth 0],[0 0 iHeight iHeight] , bg);
      | patch(logoX,logoY , fg);
      | port_label('input',1,'din');
      | port_label('input',2,'cin');
      | port_label('input',3,'msb');
      | port_label('output',1,'dout');
      | port_label('output',2,'sum');
      | port_label('output',3,'latch');
      | plot([0 0 iWidth iWidth 0], [0 iHeight iHeight 0 0]);
  Shift14 : Subsystem  mask(Normalize Shift Stage){num_bits=num_bits, bin_point=bin_point}
      mask prompts: num_bits "Number of Bits"; bin_point "Binary Point Position"
      mask init:
      | [bg,fg] = xlcmap('XBlock',0);
      | iPos = get_param(gcb,'Position');
      | iWidth=iPos(3)-iPos(1); iHeight=iPos(4)-iPos(2);
      | iCx=iWidth/2;
      | iCy=iHeight/2;
      | [logoX, logoY] = xlogo(iPos);
      mask Display:
      | patch([0 iWidth iWidth 0],[0 0 iHeight iHeight] , bg);
      | patch(logoX,logoY , fg);
      | port_label('input',1,'din');
      | port_label('input',2,'cin');
      | port_label('input',3,'msb');
      | port_label('output',1,'dout');
      | port_label('output',2,'sum');
      | port_label('output',3,'latch');
      | plot([0 0 iWidth iWidth 0], [0 iHeight iHeight 0 0]);
  Shift15 : Subsystem  mask(Normalize Shift Stage){num_bits=num_bits, bin_point=bin_point}
      mask prompts: num_bits "Number of Bits"; bin_point "Binary Point Position"
      mask init:
      | [bg,fg] = xlcmap('XBlock',0);
      | iPos = get_param(gcb,'Position');
      | iWidth=iPos(3)-iPos(1); iHeight=iPos(4)-iPos(2);
      | iCx=iWidth/2;
      | iCy=iHeight/2;
      | [logoX, logoY] = xlogo(iPos);
      mask Display:
      | patch([0 iWidth iWidth 0],[0 0 iHeight iHeight] , bg);
      | patch(logoX,logoY , fg);
      | port_label('input',1,'din');
      | port_label('input',2,'cin');
      | port_label('input',3,'msb');
      | port_label('output',1,'dout');
      | port_label('output',2,'sum');
      | port_label('output',3,'latch');
      | plot([0 0 iWidth iWidth 0], [0 iHeight iHeight 0 0]);
  Shift16 : Subsystem  mask(Normalize Shift Stage){num_bits=num_bits, bin_point=bin_point}
      mask prompts: num_bits "Number of Bits"; bin_point "Binary Point Position"
      mask init:
      | [bg,fg] = xlcmap('XBlock',0);
      | iPos = get_param(gcb,'Position');
      | iWidth=iPos(3)-iPos(1); iHeight=iPos(4)-iPos(2);
      | iCx=iWidth/2;
      | iCy=iHeight/2;
      | [logoX, logoY] = xlogo(iPos);
      mask Display:
      | patch([0 iWidth iWidth 0],[0 0 iHeight iHeight] , bg);
      | patch(logoX,logoY , fg);
      | port_label('input',1,'din');
      | port_label('input',2,'cin');
      | port_label('input',3,'msb');
      | port_label('output',1,'dout');
      | port_label('output',2,'sum');
      | port_label('output',3,'latch');
      | plot([0 0 iWidth iWidth 0], [0 iHeight iHeight 0 0]);
  Shift17 : Subsystem  mask(Normalize Shift Stage){num_bits=num_bits, bin_point=bin_point}
      mask prompts: num_bits "Number of Bits"; bin_point "Binary Point Position"
      mask init:
      | [bg,fg] = xlcmap('XBlock',0);
      | iPos = get_param(gcb,'Position');
      | iWidth=iPos(3)-iPos(1); iHeight=iPos(4)-iPos(2);
      | iCx=iWidth/2;
      | iCy=iHeight/2;
      | [logoX, logoY] = xlogo(iPos);
      mask Display:
      | patch([0 iWidth iWidth 0],[0 0 iHeight iHeight] , bg);
      | patch(logoX,logoY , fg);
      | port_label('input',1,'din');
      | port_label('input',2,'cin');
      | port_label('input',3,'msb');
      | port_label('output',1,'dout');
      | port_label('output',2,'sum');
      | port_label('output',3,'latch');
      | plot([0 0 iWidth iWidth 0], [0 iHeight iHeight 0 0]);
  Shift18 : Subsystem  mask(Normalize Shift Stage){num_bits=num_bits, bin_point=bin_point}
      mask prompts: num_bits "Number of Bits"; bin_point "Binary Point Position"
      mask init:
      | [bg,fg] = xlcmap('XBlock',0);
      | iPos = get_param(gcb,'Position');
      | iWidth=iPos(3)-iPos(1); iHeight=iPos(4)-iPos(2);
      | iCx=iWidth/2;
      | iCy=iHeight/2;
      | [logoX, logoY] = xlogo(iPos);
      mask Display:
      | patch([0 iWidth iWidth 0],[0 0 iHeight iHeight] , bg);
      | patch(logoX,logoY , fg);
      | port_label('input',1,'din');
      | port_label('input',2,'cin');
      | port_label('input',3,'msb');
      | port_label('output',1,'dout');
      | port_label('output',2,'sum');
      | port_label('output',3,'latch');
      | plot([0 0 iWidth iWidth 0], [0 iHeight iHeight 0 0]);
  Shift19 : Subsystem  mask(Normalize Shift Stage){num_bits=num_bits, bin_point=bin_point}
      mask prompts: num_bits "Number of Bits"; bin_point "Binary Point Position"
      mask init:
      | [bg,fg] = xlcmap('XBlock',0);
      | iPos = get_param(gcb,'Position');
      | iWidth=iPos(3)-iPos(1); iHeight=iPos(4)-iPos(2);
      | iCx=iWidth/2;
      | iCy=iHeight/2;
      | [logoX, logoY] = xlogo(iPos);
      mask Display:
      | patch([0 iWidth iWidth 0],[0 0 iHeight iHeight] , bg);
      | patch(logoX,logoY , fg);
      | port_label('input',1,'din');
      | port_label('input',2,'cin');
      | port_label('input',3,'msb');
      | port_label('output',1,'dout');
      | port_label('output',2,'sum');
      | port_label('output',3,'latch');
      | plot([0 0 iWidth iWidth 0], [0 iHeight iHeight 0 0]);
  Shift2 : Subsystem  mask(Normalize Shift Stage){num_bits=num_bits, bin_point=bin_point}
      mask prompts: num_bits "Number of Bits"; bin_point "Binary Point Position"
      mask init:
      | [bg,fg] = xlcmap('XBlock',0);
      | iPos = get_param(gcb,'Position');
      | iWidth=iPos(3)-iPos(1); iHeight=iPos(4)-iPos(2);
      | iCx=iWidth/2;
      | iCy=iHeight/2;
      | [logoX, logoY] = xlogo(iPos);
      mask Display:
      | patch([0 iWidth iWidth 0],[0 0 iHeight iHeight] , bg);
      | patch(logoX,logoY , fg);
      | port_label('input',1,'din');
      | port_label('input',2,'cin');
      | port_label('input',3,'msb');
      | port_label('output',1,'dout');
      | port_label('output',2,'sum');
      | port_label('output',3,'latch');
      | plot([0 0 iWidth iWidth 0], [0 iHeight iHeight 0 0]);
  Shift20 : Subsystem  mask(Normalize Shift Stage){num_bits=num_bits, bin_point=bin_point}
      mask prompts: num_bits "Number of Bits"; bin_point "Binary Point Position"
      mask init:
      | [bg,fg] = xlcmap('XBlock',0);
      | iPos = get_param(gcb,'Position');
      | iWidth=iPos(3)-iPos(1); iHeight=iPos(4)-iPos(2);
      | iCx=iWidth/2;
      | iCy=iHeight/2;
      | [logoX, logoY] = xlogo(iPos);
      mask Display:
      | patch([0 iWidth iWidth 0],[0 0 iHeight iHeight] , bg);
      | patch(logoX,logoY , fg);
      | port_label('input',1,'din');
      | port_label('input',2,'cin');
      | port_label('input',3,'msb');
      | port_label('output',1,'dout');
      | port_label('output',2,'sum');
      | port_label('output',3,'latch');
      | plot([0 0 iWidth iWidth 0], [0 iHeight iHeight 0 0]);
  Shift21 : Subsystem  mask(Normalize Shift Stage){num_bits=num_bits, bin_point=bin_point}
      mask prompts: num_bits "Number of Bits"; bin_point "Binary Point Position"
      mask init:
      | [bg,fg] = xlcmap('XBlock',0);
      | iPos = get_param(gcb,'Position');
      | iWidth=iPos(3)-iPos(1); iHeight=iPos(4)-iPos(2);
      | iCx=iWidth/2;
      | iCy=iHeight/2;
      | [logoX, logoY] = xlogo(iPos);
      mask Display:
      | patch([0 iWidth iWidth 0],[0 0 iHeight iHeight] , bg);
      | patch(logoX,logoY , fg);
      | port_label('input',1,'din');
      | port_label('input',2,'cin');
      | port_label('input',3,'msb');
      | port_label('output',1,'dout');
      | port_label('output',2,'sum');
      | port_label('output',3,'latch');
      | plot([0 0 iWidth iWidth 0], [0 iHeight iHeight 0 0]);
  Shift3 : Subsystem  mask(Normalize Shift Stage){num_bits=num_bits, bin_point=bin_point}
      mask prompts: num_bits "Number of Bits"; bin_point "Binary Point Position"
      mask init:
      | [bg,fg] = xlcmap('XBlock',0);
      | iPos = get_param(gcb,'Position');
      | iWidth=iPos(3)-iPos(1); iHeight=iPos(4)-iPos(2);
      | iCx=iWidth/2;
      | iCy=iHeight/2;
      | [logoX, logoY] = xlogo(iPos);
      mask Display:
      | patch([0 iWidth iWidth 0],[0 0 iHeight iHeight] , bg);
      | patch(logoX,logoY , fg);
      | port_label('input',1,'din');
      | port_label('input',2,'cin');
      | port_label('input',3,'msb');
      | port_label('output',1,'dout');
      | port_label('output',2,'sum');
      | port_label('output',3,'latch');
      | plot([0 0 iWidth iWidth 0], [0 iHeight iHeight 0 0]);
  Shift4 : Subsystem  mask(Normalize Shift Stage){num_bits=num_bits, bin_point=bin_point}
      mask prompts: num_bits "Number of Bits"; bin_point "Binary Point Position"
      mask init:
      | [bg,fg] = xlcmap('XBlock',0);
      | iPos = get_param(gcb,'Position');
      | iWidth=iPos(3)-iPos(1); iHeight=iPos(4)-iPos(2);
      | iCx=iWidth/2;
      | iCy=iHeight/2;
      | [logoX, logoY] = xlogo(iPos);
      mask Display:
      | patch([0 iWidth iWidth 0],[0 0 iHeight iHeight] , bg);
      | patch(logoX,logoY , fg);
      | port_label('input',1,'din');
      | port_label('input',2,'cin');
      | port_label('input',3,'msb');
      | port_label('output',1,'dout');
      | port_label('output',2,'sum');
      | port_label('output',3,'latch');
      | plot([0 0 iWidth iWidth 0], [0 iHeight iHeight 0 0]);
  Shift5 : Subsystem  mask(Normalize Shift Stage){num_bits=num_bits, bin_point=bin_point}
      mask prompts: num_bits "Number of Bits"; bin_point "Binary Point Position"
      mask init:
      | [bg,fg] = xlcmap('XBlock',0);
      | iPos = get_param(gcb,'Position');
      | iWidth=iPos(3)-iPos(1); iHeight=iPos(4)-iPos(2);
      | iCx=iWidth/2;
      | iCy=iHeight/2;
      | [logoX, logoY] = xlogo(iPos);
      mask Display:
      | patch([0 iWidth iWidth 0],[0 0 iHeight iHeight] , bg);
      | patch(logoX,logoY , fg);
      | port_label('input',1,'din');
      | port_label('input',2,'cin');
      | port_label('input',3,'msb');
      | port_label('output',1,'dout');
      | port_label('output',2,'sum');
      | port_label('output',3,'latch');
      | plot([0 0 iWidth iWidth 0], [0 iHeight iHeight 0 0]);
  Shift6 : Subsystem  mask(Normalize Shift Stage){num_bits=num_bits, bin_point=bin_point}
      mask prompts: num_bits "Number of Bits"; bin_point "Binary Point Position"
      mask init:
      | [bg,fg] = xlcmap('XBlock',0);
      | iPos = get_param(gcb,'Position');
      | iWidth=iPos(3)-iPos(1); iHeight=iPos(4)-iPos(2);
      | iCx=iWidth/2;
      | iCy=iHeight/2;
      | [logoX, logoY] = xlogo(iPos);
      mask Display:
      | patch([0 iWidth iWidth 0],[0 0 iHeight iHeight] , bg);
      | patch(logoX,logoY , fg);
      | port_label('input',1,'din');
      | port_label('input',2,'cin');
      | port_label('input',3,'msb');
      | port_label('output',1,'dout');
      | port_label('output',2,'sum');
      | port_label('output',3,'latch');
      | plot([0 0 iWidth iWidth 0], [0 iHeight iHeight 0 0]);
  Shift7 : Subsystem  mask(Normalize Shift Stage){num_bits=num_bits, bin_point=bin_point}
      mask prompts: num_bits "Number of Bits"; bin_point "Binary Point Position"
      mask init:
      | [bg,fg] = xlcmap('XBlock',0);
      | iPos = get_param(gcb,'Position');
      | iWidth=iPos(3)-iPos(1); iHeight=iPos(4)-iPos(2);
      | iCx=iWidth/2;
      | iCy=iHeight/2;
      | [logoX, logoY] = xlogo(iPos);
      mask Display:
      | patch([0 iWidth iWidth 0],[0 0 iHeight iHeight] , bg);
      | patch(logoX,logoY , fg);
      | port_label('input',1,'din');
      | port_label('input',2,'cin');
      | port_label('input',3,'msb');
      | port_label('output',1,'dout');
      | port_label('output',2,'sum');
      | port_label('output',3,'latch');
      | plot([0 0 iWidth iWidth 0], [0 iHeight iHeight 0 0]);
  Shift8 : Subsystem  mask(Normalize Shift Stage){num_bits=num_bits, bin_point=bin_point}
      mask prompts: num_bits "Number of Bits"; bin_point "Binary Point Position"
      mask init:
      | [bg,fg] = xlcmap('XBlock',0);
      | iPos = get_param(gcb,'Position');
      | iWidth=iPos(3)-iPos(1); iHeight=iPos(4)-iPos(2);
      | iCx=iWidth/2;
      | iCy=iHeight/2;
      | [logoX, logoY] = xlogo(iPos);
      mask Display:
      | patch([0 iWidth iWidth 0],[0 0 iHeight iHeight] , bg);
      | patch(logoX,logoY , fg);
      | port_label('input',1,'din');
      | port_label('input',2,'cin');
      | port_label('input',3,'msb');
      | port_label('output',1,'dout');
      | port_label('output',2,'sum');
      | port_label('output',3,'latch');
      | plot([0 0 iWidth iWidth 0], [0 iHeight iHeight 0 0]);
  Shift9 : Subsystem  mask(Normalize Shift Stage){num_bits=num_bits, bin_point=bin_point}
      mask prompts: num_bits "Number of Bits"; bin_point "Binary Point Position"
      mask init:
      | [bg,fg] = xlcmap('XBlock',0);
      | iPos = get_param(gcb,'Position');
      | iWidth=iPos(3)-iPos(1); iHeight=iPos(4)-iPos(2);
      | iCx=iWidth/2;
      | iCy=iHeight/2;
      | [logoX, logoY] = xlogo(iPos);
      mask Display:
      | patch([0 iWidth iWidth 0],[0 0 iHeight iHeight] , bg);
      | patch(logoX,logoY , fg);
      | port_label('input',1,'din');
      | port_label('input',2,'cin');
      | port_label('input',3,'msb');
      | port_label('output',1,'dout');
      | port_label('output',2,'sum');
      | port_label('output',3,'latch');
      | plot([0 0 iWidth iWidth 0], [0 iHeight iHeight 0 0]);
  Terminator1 : Terminator
  norm : Outport  OutDataType=sfix(16)  OutScaling=2^0
  shift : Outport  Port=2  OutDataType=sfix(16)  OutScaling=2^0
  wires:
  msb/1 -> Shift1/3(msb)
  cin/1 -> Shift1/2(cin)
  abs/1 -> Shift1/1(din)
  Shift1/1(dout) -> Shift2/1(din)
  Shift1/2(sum) -> Shift2/2(cin)
  Shift1/3(latch) -> Shift2/3(msb)
  Shift2/1(dout) -> Shift3/1(din)
  Shift2/2(sum) -> Shift3/2(cin)
  Shift2/3(latch) -> Shift3/3(msb)
  Shift3/1(dout) -> Shift4/1(din)
  Shift3/2(sum) -> Shift4/2(cin)
  Shift3/3(latch) -> Shift4/3(msb)
  Shift4/1(dout) -> Shift5/1(din)
  Shift4/2(sum) -> Shift5/2(cin)
  Shift4/3(latch) -> Shift5/3(msb)
  Shift5/1(dout) -> Shift6/1(din)
  Shift5/2(sum) -> Shift6/2(cin)
  Shift5/3(latch) -> Shift6/3(msb)
  Shift6/1(dout) -> Shift7/1(din)
  Shift6/2(sum) -> Shift7/2(cin)
  Shift6/3(latch) -> Shift7/3(msb)
  Shift7/1(dout) -> Shift8/1(din)
  Shift7/2(sum) -> Shift8/2(cin)
  Shift7/3(latch) -> Shift8/3(msb)
  Shift8/1(dout) -> Shift9/1(din)
  Shift8/2(sum) -> Shift9/2(cin)
  Shift8/3(latch) -> Shift9/3(msb)
  Shift9/1(dout) -> Shift10/1(din)
  Shift9/2(sum) -> Shift10/2(cin)
  Shift9/3(latch) -> Shift10/3(msb)
  Shift10/1(dout) -> Shift11/1(din)
  Shift10/2(sum) -> Shift11/2(cin)
  Shift10/3(latch) -> Shift11/3(msb)
  Shift11/1(dout) -> Shift12/1(din)
  Shift11/2(sum) -> Shift12/2(cin)
  Shift11/3(latch) -> Shift12/3(msb)
  Shift12/1(dout) -> Shift13/1(din)
  Shift12/2(sum) -> Shift13/2(cin)
  Shift12/3(latch) -> Shift13/3(msb)
  Shift13/1(dout) -> Shift14/1(din)
  Shift13/2(sum) -> Shift14/2(cin)
  Shift13/3(latch) -> Shift14/3(msb)
  Shift14/1(dout) -> Shift15/1(din)
  Shift14/2(sum) -> Shift15/2(cin)
  Shift14/3(latch) -> Shift15/3(msb)
  Shift15/1(dout) -> Shift16/1(din)
  Shift15/2(sum) -> Shift16/2(cin)
  Shift15/3(latch) -> Shift16/3(msb)
  Shift16/1(dout) -> Shift17/1(din)
  Shift16/2(sum) -> Shift17/2(cin)
  Shift16/3(latch) -> Shift17/3(msb)
  Shift17/1(dout) -> Shift18/1(din)
  Shift17/2(sum) -> Shift18/2(cin)
  Shift17/3(latch) -> Shift18/3(msb)
  Shift18/1(dout) -> Shift19/1(din)
  Shift18/2(sum) -> Shift19/2(cin)
  Shift18/3(latch) -> Shift19/3(msb)
  Shift19/1(dout) -> Shift20/1(din)
  Shift19/2(sum) -> Shift20/2(cin)
  Shift19/3(latch) -> Shift20/3(msb)
  Shift20/1(dout) -> Shift21/1(din)
  Shift20/2(sum) -> Shift21/2(cin)
  Shift20/3(latch) -> Shift21/3(msb)
  Shift21/1(dout) -> norm/1
  Shift21/2(sum) -> shift/1
  Shift21/3(latch) -> Terminator1/1
